simulink model "Modelo_global_NL_2_a_II"  (R2017a)
settings: Solver=VariableStepAuto  StartTime=0.0  StopTime=10.0  RelTol=1e-3
undefined symbols (not defined in the file): alfa_cu, beq, Cts, Jeq, LambdaM, Ld, Lq, Pp, Rs, Rsref, Rts, Tamb, Tsref
libraries: simulink x3
settings Model: Creator=merem  LastModifiedBy=merem

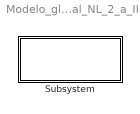
== system Modelo_global_NL_2_a_II ==
  Subsystem : Subsystem

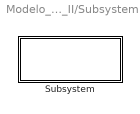
== system Modelo_global_NL_2_a_II/Subsystem ==
  Subsystem : Subsystem

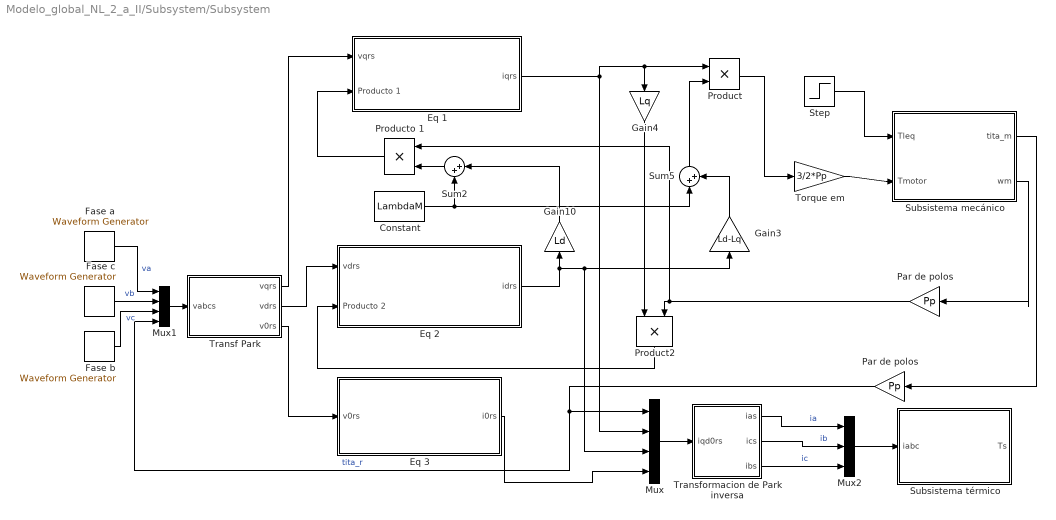
== system Modelo_global_NL_2_a_II/Subsystem/Subsystem ==
  Constant : Constant  Value=LambdaM
  Eq 1 : Subsystem
  "Eq 2 " : Subsystem
  Eq 3 : Subsystem
  "Fase a " : simulink/Sources/Waveform Generator  OutMin=[]  OutMax=[]  OutDataTypeStr=double  SelectedSignal=1  BlockNames=MultiportSwitch_e3df3653d217406  SampleTime=0.1
      settings: SourceProductName=Simulink
  "Fase b " : simulink/Sources/Waveform Generator  OutMin=[]  OutMax=[]  OutDataTypeStr=double  SelectedSignal=1  BlockNames=MultiportSwitch_e3df3653d217406  SampleTime=0.1
      settings: SourceProductName=Simulink
  Fase c : simulink/Sources/Waveform Generator  OutMin=[]  OutMax=[]  OutDataTypeStr=double  SelectedSignal=1  BlockNames=MultiportSwitch_e3df3653d217406  SampleTime=0.1
      settings: SourceProductName=Simulink
  Gain10 : Gain  Gain=Ld
  Gain3 : Gain  Gain=Ld-Lq
  Gain4 : Gain  Gain=Lq
  Mux : Mux
  Mux1 : Mux
  Mux2 : Mux  Inputs=3
  Par de polos : Gain  Gain=Pp
  "Par de polos " : Gain  Gain=Pp
  Product : Product
  Product2 : Product
  Producto 1 : Product
  Step : Step  After=6.28  SampleTime=0
  Subsistema mecánico : Subsystem
  Subsistema térmico : Subsystem
  Sum2 : Sum  Inputs=|++
  Sum5 : Sum  Inputs=|++
  "Torque em " : Gain  Gain=3/2*Pp
  "Transf Park " : Subsystem
  "Transformacion de Park inversa " : Subsystem
  wires:
  Product/1 -> "Torque em "/1
  Par de polos/1 -> Product2/2, Producto 1/1
  Sum2/1 -> Producto 1/2
  Gain10/1 -> Sum2/1
  Constant/1 -> Sum5/1, Sum2/2
  Sum5/1 -> Product/2
  Gain3/1 -> Sum5/2
  Gain4/1 -> Product2/1
  Eq 1/1("iqrs ") -> Gain4/1, Product/1, Mux/2
  Producto 1/1 -> Eq 1/2("Producto 1 ")
  "Eq 2 "/1("idrs ") -> Mux/3, Gain3/1, Gain10/1
  Product2/1 -> "Eq 2 "/2("Producto 2 ")
  Step/1 -> Subsistema mecánico/1("Tleq ")
  "Torque em "/1 -> Subsistema mecánico/2("Tmotor ")
  Subsistema mecánico/2("wm ") -> Par de polos/1
  Subsistema mecánico/1("tita_m ") -> "Par de polos "/1
  "Par de polos "/1 -> Mux/1, Mux1/4  "tita_r"
  "Transf Park "/1(vqrs) -> Eq 1/1(vqrs)
  "Transf Park "/2("vdrs ") -> "Eq 2 "/1("vdrs ")
  "Transf Park "/3("v0rs ") -> Eq 3/1("v0rs ")
  Mux/1 -> "Transformacion de Park inversa "/1(iqd0rs)
  "Fase a "/1 -> Mux1/1  "va"
  Fase c/1 -> Mux1/2  "vb"
  "Fase b "/1 -> Mux1/3  "vc"
  Mux1/1 -> "Transf Park "/1("vabcs ")
  Eq 3/1("i0rs ") -> Mux/4
  Mux2/1 -> Subsistema térmico/1(iabc)
  "Transformacion de Park inversa "/1(ias) -> Mux2/1  "ia"
  "Transformacion de Park inversa "/2("ics ") -> Mux2/2  "ib"
  "Transformacion de Park inversa "/3(ibs) -> Mux2/3  "ic"

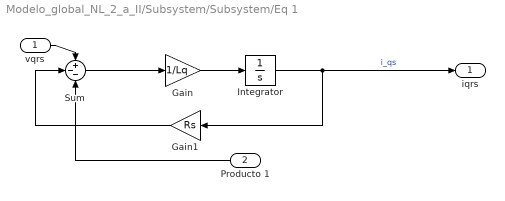
== system Modelo_global_NL_2_a_II/Subsystem/Subsystem/Eq 1 ==
  vqrs : Inport
  "Producto 1 " : Inport  Port=2
  Gain : Gain  Gain=1/Lq
  Gain1 : Gain  Gain=Rs
  Integrator : Integrator
  Sum : Sum  Inputs=+--
  "iqrs " : Outport
  wires:
  Gain/1 -> Integrator/1
  Sum/1 -> Gain/1
  vqrs/1 -> Sum/1
  Gain1/1 -> Sum/2
  "Producto 1 "/1 -> Sum/3
  Integrator/1 -> "iqrs "/1, Gain1/1  "i_qs"

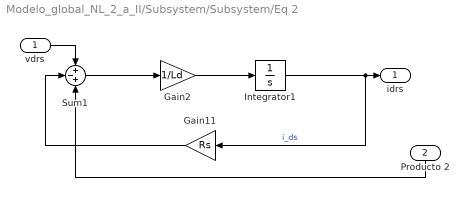
== system Modelo_global_NL_2_a_II/Subsystem/Subsystem/Eq 2  ==
  "vdrs " : Inport
  "Producto 2 " : Inport  Port=2
  Gain11 : Gain  Gain=Rs
  Gain2 : Gain  Gain=1/Ld
  Integrator1 : Integrator
  Sum1 : Sum  Inputs=+-+
  "idrs " : Outport
  wires:
  "Producto 2 "/1 -> Sum1/3
  Gain2/1 -> Integrator1/1
  Gain11/1 -> Sum1/2
  Sum1/1 -> Gain2/1
  Integrator1/1 -> Gain11/1, "idrs "/1  "i_ds"
  "vdrs "/1 -> Sum1/1

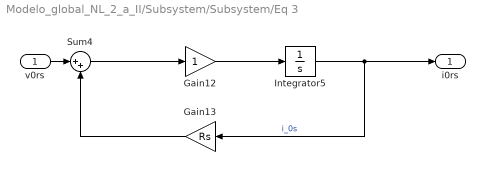
== system Modelo_global_NL_2_a_II/Subsystem/Subsystem/Eq 3 ==
  "v0rs " : Inport
  Gain12 : Gain
  Gain13 : Gain  Gain=Rs
  Integrator5 : Integrator
  Sum4 : Sum  Inputs=|++
  "i0rs " : Outport
  wires:
  Gain12/1 -> Integrator5/1
  Sum4/1 -> Gain12/1
  Gain13/1 -> Sum4/2
  "v0rs "/1 -> Sum4/1
  Integrator5/1 -> "i0rs "/1, Gain13/1  "i_0s"

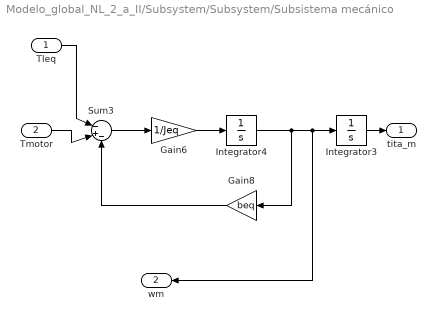
== system Modelo_global_NL_2_a_II/Subsystem/Subsystem/Subsistema mecánico ==
  "Tleq " : Inport
  "Tmotor " : Inport  Port=2
  Gain6 : Gain  Gain=1/Jeq
  Gain8 : Gain  Gain=beq
  Integrator3 : Integrator
  Integrator4 : Integrator
  Sum3 : Sum  Inputs=|-+-
  "tita_m " : Outport
  "wm " : Outport  Port=2
  wires:
  Integrator3/1 -> "tita_m "/1
  Integrator4/1 -> Gain8/1, "wm "/1, Integrator3/1
  Sum3/1 -> Gain6/1
  Gain6/1 -> Integrator4/1
  Gain8/1 -> Sum3/3
  "Tleq "/1 -> Sum3/1
  "Tmotor "/1 -> Sum3/2

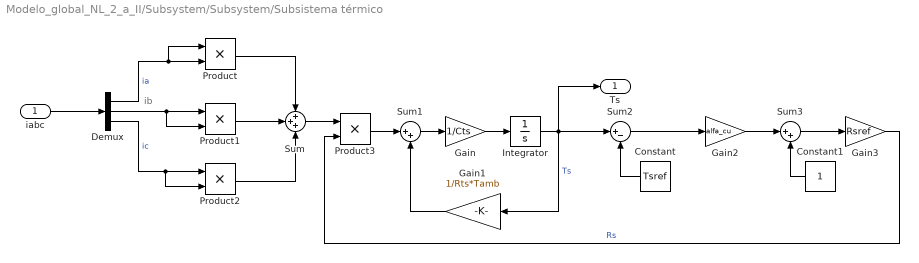
== system Modelo_global_NL_2_a_II/Subsystem/Subsystem/Subsistema térmico ==
  note: ib
  iabc : Inport
  Constant : Constant  Value=Tsref
  Constant1 : Constant
  Demux : Demux  Outputs=3
  Gain : Gain  Gain=1/Cts
  Gain1 : Gain  Gain=1/Rts*Tamb
  Gain2 : Gain  Gain=alfa_cu
  Gain3 : Gain  Gain=Rsref
  Integrator : Integrator
  Product{,1..3} (4 alike) : Product
  Sum : Sum  Inputs=+++
  Sum1 : Sum  Inputs=|++
  Sum2 : Sum  Inputs=|+-
  Sum3 : Sum  Inputs=|++
  Ts : Outport
  wires:
  iabc/1 -> Demux/1
  Demux/1 -> Product/2, Product/1  "ia"
  Demux/2 -> Product1/2, Product1/1
  Demux/3 -> Product2/2, Product2/1  "ic"
  Product/1 -> Sum/1
  Product1/1 -> Sum/2
  Product2/1 -> Sum/3
  Sum/1 -> Product3/1
  Gain/1 -> Integrator/1
  Product3/1 -> Sum1/1
  Sum1/1 -> Gain/1
  Gain1/1 -> Sum1/2
  Integrator/1 -> Ts/1, Sum2/1, Gain1/1  "Ts"
  Constant/1 -> Sum2/2
  Sum2/1 -> Gain2/1
  Gain2/1 -> Sum3/1
  Constant1/1 -> Sum3/2
  Sum3/1 -> Gain3/1
  Gain3/1 -> Product3/2  "Rs"

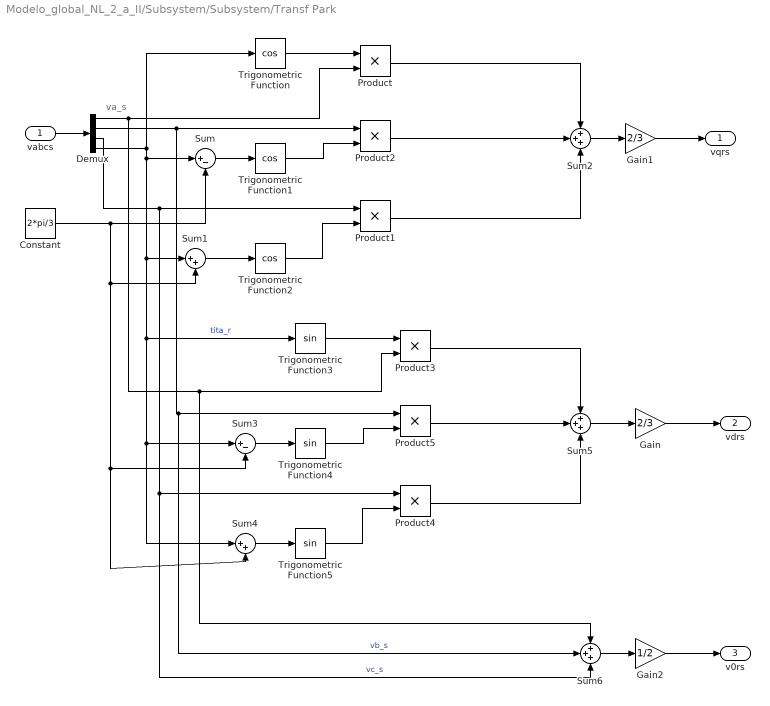
== system Modelo_global_NL_2_a_II/Subsystem/Subsystem/Transf Park  ==
  note: va_s
  "vabcs " : Inport
  Constant : Constant  Value=2*pi/3
  Demux : Demux
  Gain : Gain  Gain=2/3
  Gain1 : Gain  Gain=2/3
  Gain2 : Gain  Gain=1/2
  Product{,1..5} (6 alike) : Product
  Sum : Sum  Inputs=|+-
  Sum1 : Sum  Inputs=|++
  Sum2 : Sum  Inputs=+++
  Sum3 : Sum  Inputs=|+-
  Sum4 : Sum  Inputs=|++
  Sum5 : Sum  Inputs=+++
  Sum6 : Sum  Inputs=+++
  Trigonometric Function : Trigonometry  Operator=cos
  Trigonometric Function1 : Trigonometry  Operator=cos
  Trigonometric Function2 : Trigonometry  Operator=cos
  Trigonometric Function3 : Trigonometry
  Trigonometric Function4 : Trigonometry
  Trigonometric Function5 : Trigonometry
  vqrs : Outport
  "vdrs " : Outport  Port=2
  "v0rs " : Outport  Port=3
  wires:
  "vabcs "/1 -> Demux/1
  Demux/4 -> Sum1/1, Trigonometric Function3/1, Sum3/1, Sum4/1, Sum/1, Trigonometric Function/1  "tita_r"
  Trigonometric Function/1 -> Product/1
  Demux/1 -> Sum6/1, Product3/2, Product/2
  Constant/1 -> Sum4/2, Sum3/2, Sum1/2, Sum/2
  Sum/1 -> Trigonometric Function1/1
  Sum1/1 -> Trigonometric Function2/1
  Trigonometric Function1/1 -> Product2/2
  Trigonometric Function2/1 -> Product1/2
  Demux/2 -> Sum6/2, Product5/1, Product2/1  "vb_s"
  Demux/3 -> Sum6/3, Product4/1, Product1/1  "vc_s"
  Product/1 -> Sum2/1
  Product2/1 -> Sum2/2
  Sum2/1 -> Gain1/1
  Trigonometric Function5/1 -> Product4/2
  Trigonometric Function3/1 -> Product3/1
  Sum4/1 -> Trigonometric Function5/1
  Sum3/1 -> Trigonometric Function4/1
  Trigonometric Function4/1 -> Product5/2
  Product3/1 -> Sum5/1
  Product5/1 -> Sum5/2
  Product4/1 -> Sum5/3
  Sum5/1 -> Gain/1
  Product1/1 -> Sum2/3
  Gain/1 -> "vdrs "/1
  Gain1/1 -> vqrs/1
  Sum6/1 -> Gain2/1
  Gain2/1 -> "v0rs "/1

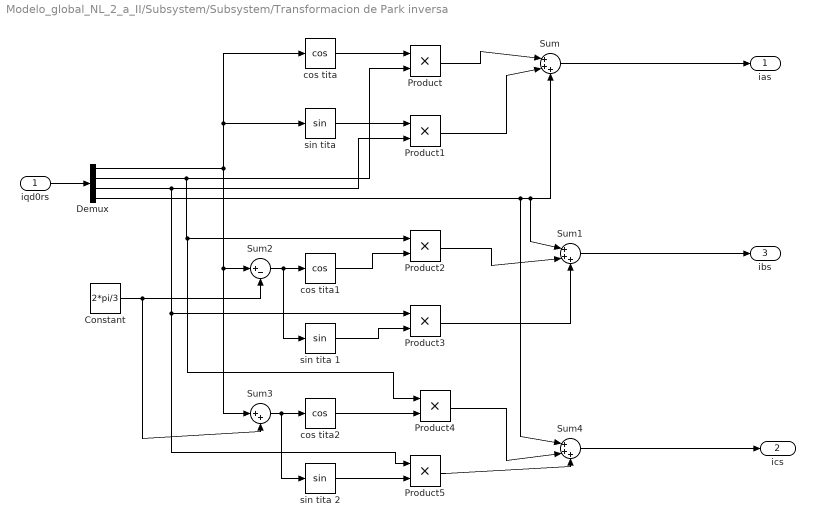
== system Modelo_global_NL_2_a_II/Subsystem/Subsystem/Transformacion de Park inversa  ==
  iqd0rs : Inport
  Constant : Constant  Value=2*pi/3
  Demux : Demux
  Product{,1..5} (6 alike) : Product
  Sum : Sum  Inputs=|+++
  Sum1 : Sum  Inputs=|+++
  Sum2 : Sum  Inputs=|+-
  Sum3 : Sum  Inputs=|++
  Sum4 : Sum  Inputs=|+++
  cos tita : Trigonometry  Operator=cos
  cos tita1 : Trigonometry  Operator=cos
  cos tita2 : Trigonometry  Operator=cos
  "sin tita " : Trigonometry
  sin tita 1 : Trigonometry
  sin tita 2 : Trigonometry
  ias : Outport
  "ics " : Outport  Port=2
  ibs : Outport  Port=3
  wires:
  iqd0rs/1 -> Demux/1
  Demux/1 -> Sum3/1, Sum2/1, cos tita/1, "sin tita "/1
  Demux/2 -> Product4/1, Product2/1, Product/2
  cos tita/1 -> Product/1
  "sin tita "/1 -> Product1/1
  Demux/3 -> Product5/1, Product3/1, Product1/2
  Product/1 -> Sum/1
  Product1/1 -> Sum/2
  Sum/1 -> ias/1
  Demux/4 -> Sum4/1, Sum1/1, Sum/3
  cos tita1/1 -> Product2/2
  sin tita 1/1 -> Product3/2
  Product3/1 -> Sum1/3
  Product2/1 -> Sum1/2
  Sum1/1 -> ibs/1
  Constant/1 -> Sum3/2, Sum2/2
  Sum2/1 -> sin tita 1/1, cos tita1/1
  Sum3/1 -> sin tita 2/1, cos tita2/1
  cos tita2/1 -> Product4/2
  sin tita 2/1 -> Product5/2
  Product5/1 -> Sum4/3
  Product4/1 -> Sum4/2
  Sum4/1 -> "ics "/1
